simulink model "questao2"  (R2023a)
settings: Solver=VariableStepAuto  StartTime=0.0  StopTime=125  RelTol=1e-3
values from neighbouring files (symbols this model uses):
  B = 0.1    [trab_controle.m]
  J = 1    [trab_controle.m]
  Km = 1/3    (= 0.333333333333)    [trab_controle.m]
  L = 0.5    [trab_controle.m]
  R = 10    [trab_controle.m]
settings Model: Creator=Maria  LastModifiedBy=franz

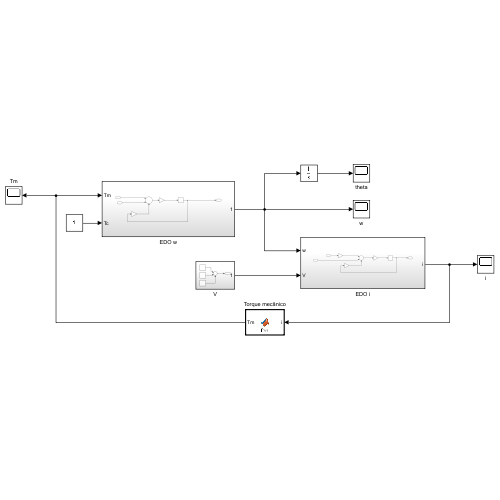
[thumbnail: Simulink's stored preview of the top-level diagram]
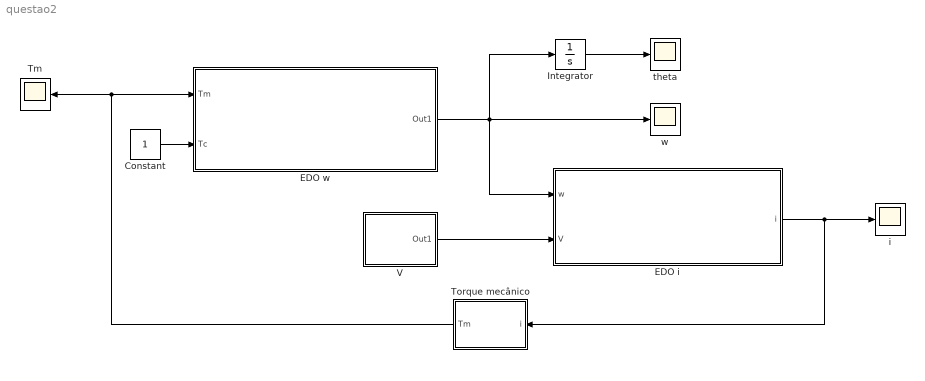
== system questao2 ==
  Constant : Constant
  EDO i : Subsystem
  EDO w : Subsystem
  Integrator : Integrator
  Tm : Scope
  Torque mecânico : MATLAB Function  TreatAsAtomicUnit=on
  V : Subsystem
  i : Scope
  theta : Scope
  w : Scope
  wires:
  Torque mecânico/1(Tm) -> Tm/1, EDO w/1(Tm)
  EDO w/1(Out1) -> Integrator/1, EDO i/1(w), w/1
  EDO i/1(i) -> Torque mecânico/1(i), i/1
  Integrator/1 -> theta/1
  Constant/1 -> EDO w/2(Tc)
  V/1(Out1) -> EDO i/2(V)

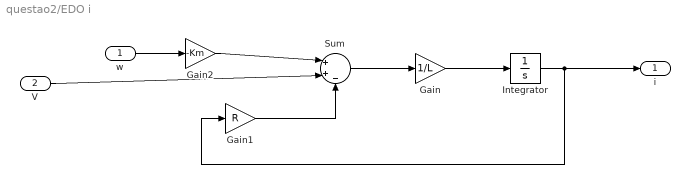
== system questao2/EDO i ==
  w : Inport
  V : Inport  Port=2
  Gain : Gain  Gain=1/L
  Gain1 : Gain  Gain=R
  Gain2 : Gain  Gain=-Km
  Integrator : Integrator
  Sum : Sum  Inputs=|++-
  i : Outport
  wires:
  Gain1/1 -> Sum/3
  Integrator/1 -> i/1, Gain1/1
  Gain/1 -> Integrator/1
  Sum/1 -> Gain/1
  V/1 -> Sum/2
  w/1 -> Gain2/1
  Gain2/1 -> Sum/1

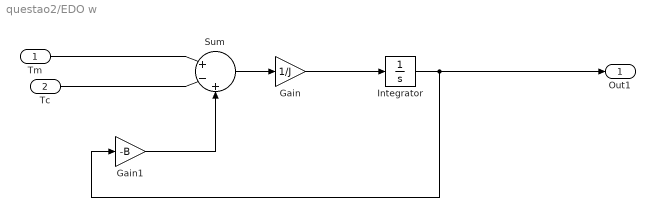
== system questao2/EDO w ==
  Tm : Inport
  Tc : Inport  Port=2
  Gain : Gain  Gain=1/J
  Gain1 : Gain  Gain=-B
  Integrator : Integrator
  Sum : Sum  Inputs=|+-+
  Out1 : Outport
  wires:
  Integrator/1 -> Out1/1, Gain1/1
  Gain1/1 -> Sum/3
  Gain/1 -> Integrator/1
  Tc/1 -> Sum/2
  Sum/1 -> Gain/1
  Tm/1 -> Sum/1

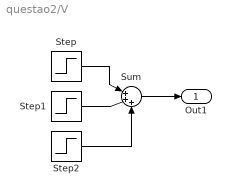
== system questao2/V ==
  Step : Step  Time=25  Before=20  After=21  SampleTime=0
  Step1 : Step  Time=50  After=0  SampleTime=0
  Step2 : Step  Time=75  After=0  SampleTime=0
  Sum : Sum  Inputs=|+++
  Out1 : Outport
  wires:
  Step1/1 -> Sum/2
  Step2/1 -> Sum/3
  Step/1 -> Sum/1
  Sum/1 -> Out1/1

== matlab function questao2/Torque mecânico ==
  data: i input; Tm output
function Tm = fcn(i)

if i >= 0
    torque_m = 5.26*(1 - exp(-i));
else
    torque_m = -5.26*(1 - exp(i));
end


Tm = torque_m;
